simulink subsystem "tehrani_alv_mass_balance v2"  (R2019b)
settings: Solver=VariableStepAuto  StartTime=0.0  StopTime=10.0  RelTol=1e-3
settings Model: Creator=RH  LastModifiedBy=RH

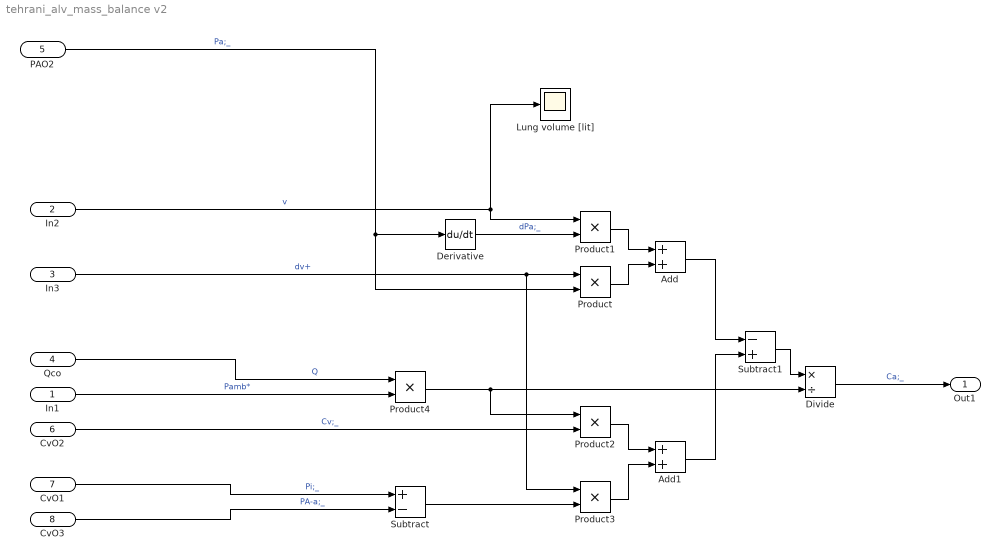
== system tehrani_alv_mass_balance v2 ==
  In1 : Inport
  In2 : Inport  Port=2
  In3 : Inport  Port=3
  Qco : Inport  Port=4
  PAO2 : Inport  Port=5
  CvO2 : Inport  Port=6
  CvO1 : Inport  Port=7
  CvO3 : Inport  Port=8
  Add : Sum
  Add1 : Sum
  Derivative : Derivative
  Divide : Product  Inputs=*/
  Lung volume [lit] : Scope
  Product{,1..4} (5 alike) : Product
  Subtract : Sum  Inputs=+-
  Subtract1 : Sum  Inputs=-+
  Out1 : Outport
  wires:
  CvO2/1 -> Product2/2  "Cv;_"
  Divide/1 -> Out1/1  "Ca;_"
  Qco/1 -> Product4/1  "Q"
  In1/1 -> Product4/2  "Pamb*"
  Product1/1 -> Add/1
  Derivative/1 -> Product1/2  "dPa;_"
  In2/1 -> Product1/1, Lung volume [lit]/1  "v"
  PAO2/1 -> Derivative/1, Product/2  "Pa;_"
  Product/1 -> Add/2
  CvO1/1 -> Subtract/1  "Pi;_"
  CvO3/1 -> Subtract/2  "PA-a;_"
  Subtract/1 -> Product3/2
  Product3/1 -> Add1/2
  Add1/1 -> Subtract1/2
  Add/1 -> Subtract1/1
  Product4/1 -> Divide/2, Product2/1
  Product2/1 -> Add1/1
  Subtract1/1 -> Divide/1
  In3/1 -> Product/1, Product3/1  "dv+"
